simulink model "test2"  (R2020b)
settings: Solver=VariableStepAuto  StartTime=0.0  StopTime=50  RelTol=1e-3
values from neighbouring files (symbols this model uses):
  A = [-18/7 9 0;1 -1 1;0 -14.28 0]    [test2.m]
  C = [1 0 0]    [test2.m]
  H = [27/7;0;0]    [test2.m]
settings Model: Creator=10911  LastModifiedBy=10911

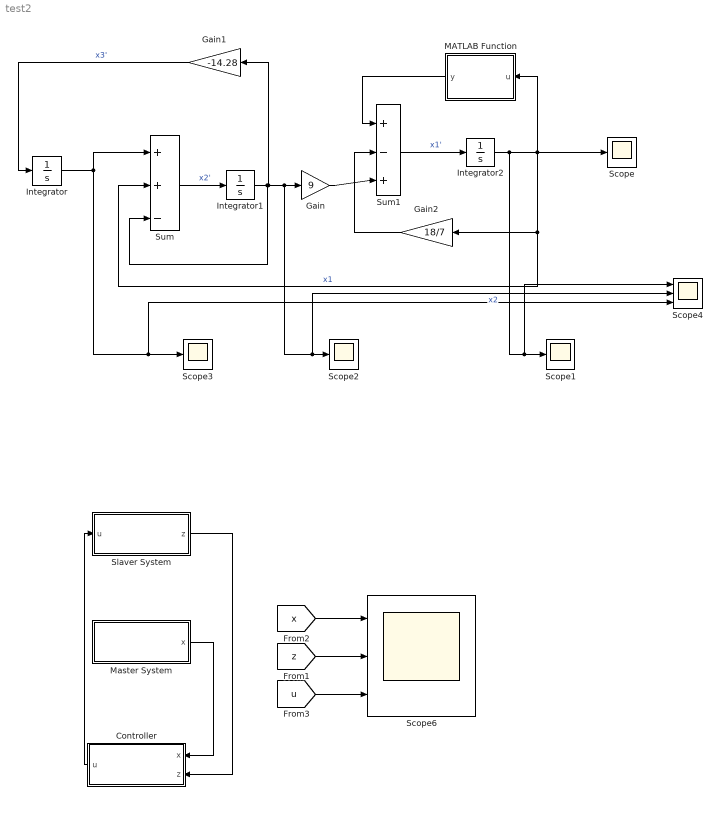
== system test2 ==
  Controller : Subsystem
  Gain : Gain  Gain=9
  Gain1 : Gain  Gain=-14.28
  Gain2 : Gain  Gain=18/7
  Integrator : Integrator  InitialCondition=0.2
  Integrator1 : Integrator  InitialCondition=0.1
  Integrator2 : Integrator  InitialCondition=-0.1
  MATLAB Function : MATLAB Function  TreatAsAtomicUnit=on
  Master System : Subsystem
  Scope{,1..3} (4 alike) : Scope
  Scope4 : Scope  NumInputPorts=3
  Scope6 : Scope  NumInputPorts=3
  Slaver System : Subsystem
  Sum : Sum  Inputs=|++-
  Sum1 : Sum  Inputs=|+-+
  wires:
  Integrator/1 -> Scope4/3, Scope3/1, Sum/1
  MATLAB Function/1(y) -> Sum1/1
  Integrator2/1 -> Scope4/1, Scope1/1, MATLAB Function/1(u), Scope/1, Gain2/1, Sum/2  "x1"
  Gain2/1 -> Sum1/2
  Gain/1 -> Sum1/3
  Sum1/1 -> Integrator2/1  "x1'"
  Gain1/1 -> Integrator/1  "x3'"
  Integrator1/1 -> Sum/3, Scope4/2, Scope2/1, Gain/1, Gain1/1  "x2"
  Sum/1 -> Integrator1/1  "x2'"
  Controller/1(u) -> Slaver System/1(u)
  Master System/1(x) -> Controller/1(x)
  Slaver System/1(z) -> Controller/2(z)
  [x] -> Scope6/1
  [z] -> Scope6/2
  [u] -> Scope6/3

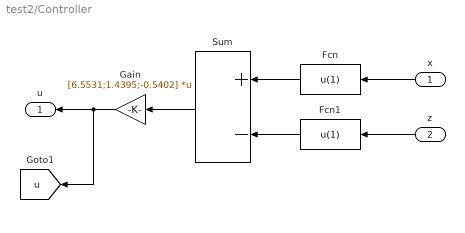
== system test2/Controller ==
  x : Inport
  z : Inport  Port=2
  Fcn : Fcn  Expr=u(1)
  Fcn1 : Fcn  Expr=u(1)
  Gain : Gain  Gain=[6.5531;1.4395;-0.5402]  Multiplication=Matrix(K*u)
  Sum : Sum  Inputs=+-
  u : Outport
  tag scope: u=global
  wires:
  z/1 -> Fcn1/1
  x/1 -> Fcn/1
  Fcn/1 -> Sum/1
  Fcn1/1 -> Sum/2
  Sum/1 -> Gain/1
  Gain/1 -> [u], u/1

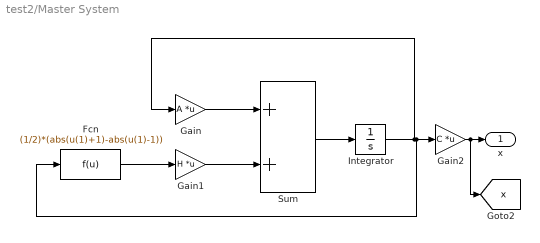
== system test2/Master System ==
  Fcn : Fcn  Expr=(1/2)*(abs(u(1)+1)-abs(u(1)-1))
  Gain : Gain  Gain=A  Multiplication=Matrix(K*u)
  Gain1 : Gain  Gain=H  Multiplication=Matrix(K*u)
  Gain2 : Gain  Gain=C  Multiplication=Matrix(K*u)
  Integrator : Integrator  InitialCondition=[-0.2;0.3;0.7]
  Sum : Sum
  x : Outport
  tag scope: x=global
  wires:
  Gain/1 -> Sum/1
  Gain1/1 -> Sum/2
  Sum/1 -> Integrator/1
  Integrator/1 -> Gain2/1, Fcn/1, Gain/1
  Fcn/1 -> Gain1/1
  Gain2/1 -> [x], x/1

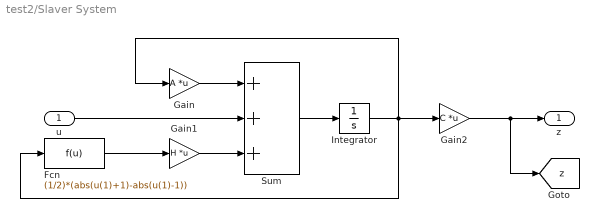
== system test2/Slaver System ==
  u : Inport
  Fcn : Fcn  Expr=(1/2)*(abs(u(1)+1)-abs(u(1)-1))
  Gain : Gain  Gain=A  Multiplication=Matrix(K*u)
  Gain1 : Gain  Gain=H  Multiplication=Matrix(K*u)
  Gain2 : Gain  Gain=C  Multiplication=Matrix(K*u)
  Integrator : Integrator  InitialCondition=[0.2;0.3;0.7]
  Sum : Sum  Inputs=+++
  z : Outport
  tag scope: z=global
  wires:
  Gain/1 -> Sum/1
  Integrator/1 -> Fcn/1, Gain2/1, Gain/1
  Sum/1 -> Integrator/1
  Fcn/1 -> Gain1/1
  Gain1/1 -> Sum/3
  u/1 -> Sum/2
  Gain2/1 -> [z], z/1

== matlab function test2/MATLAB Function ==
  data: u input; y output
function y = fcn(u)

y = 9*3/14*(abs(u+1)-abs(u-1));
